simulink model "gimbal_model_dynamics_kinematics_test_250120"  (R2018b)
settings: Solver=VariableStepAuto  StartTime=0.0  StopTime=10.0  RelTol=1e-3
values from neighbouring files (symbols this model uses):
  DIM = data{4}    [gimbal_dynamics.m]
  DIS = data{5}    [gimbal_dynamics.m]
  I1 = data{1}    [gimbal_dynamics.m]    (also in macierze_inercji.m = sym('I1', [4 4]))
  I2 = data{2}    [gimbal_dynamics.m]    (also in macierze_inercji.m = sym('I2', [4 4]))
  I3 = data{3}    [gimbal_dynamics.m]    (also in macierze_inercji.m = sym('I3', [4 4]))
  M = [ud_ucz(3:p-1) ud_ucz(3:p-1).^2 ud_ucz(3:p-1).^3 ud_ucz(2:p-2) ud_ucz(2:p-2).^2 ud_ucz(2:p-2).^3 ud_ucz(1:p-3) ud_ucz(1:p-3).^2 ud_ucz(1:p-3).^3 yd_ucz(3:p-1) yd_ucz(3:p-1).^2 yd_ucz(3:p-1).^3 yd_ucz(2:p-2) yd_ucz(2:p-2).^2 yd_ucz(2:p-2).^3 yd_ucz(1:p-3) yd_ucz(1:p-3).^2 yd_ucz(1:p-3).^3]    [Identification_20191023.m]    (also in MI_beta.m = fillmissing(M,'spline'); gimbal_dynamics.m = data{6}; macierze_inercji.m = sym('M', [1 3]))
libraries: robotcorelib x5
settings Model: Creator=Paweł Tymiński  LastModifiedBy=Paweł Tymiński

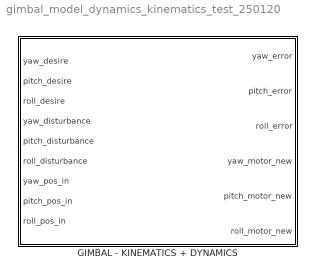
== system gimbal_model_dynamics_kinematics_test_250120 ==
  GIMBAL - KINEMATICS + DYNAMICS : Subsystem

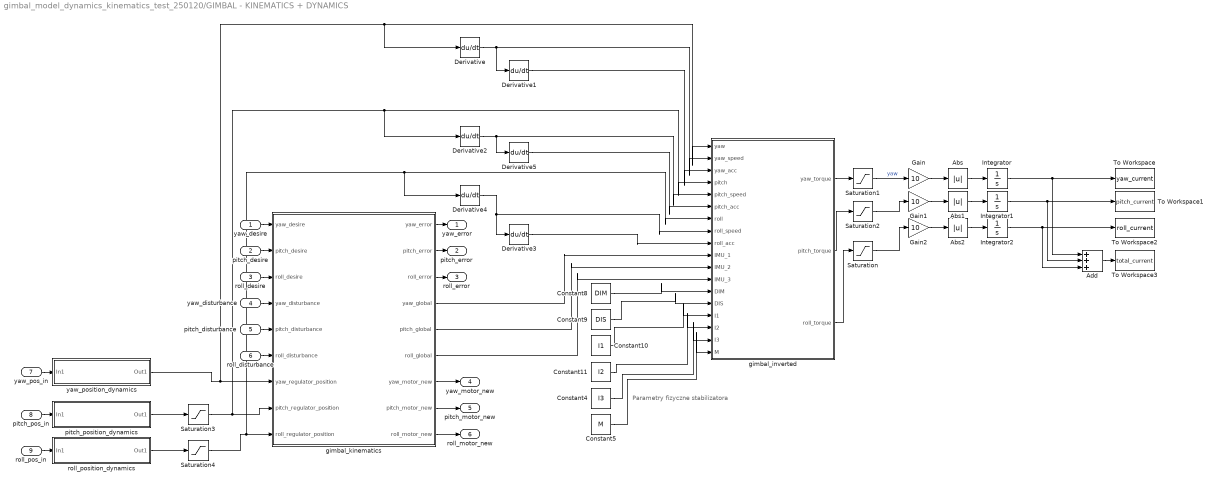
== system gimbal_model_dynamics_kinematics_test_250120/GIMBAL - KINEMATICS + DYNAMICS ==
  note: Parametry fizyczne stabilizatora
  yaw_desire : Inport
  pitch_desire : Inport  Port=2
  roll_desire : Inport  Port=3
  yaw_disturbance : Inport  Port=4
  pitch_disturbance : Inport  Port=5
  roll_disturbance : Inport  Port=6
  yaw_pos_in : Inport  Port=7
  pitch_pos_in : Inport  Port=8
  roll_pos_in : Inport  Port=9
  Abs : Abs
  Abs1 : Abs
  Abs2 : Abs
  Add : Sum  Inputs=+++
  Constant10 : Constant  Value=I1
  Constant11 : Constant  Value=I2
  Constant4 : Constant  Value=I3
  Constant5 : Constant  Value=M
  Constant8 : Constant  Value=DIM
  Constant9 : Constant  Value=DIS
  Derivative{,1..5} (6 alike) : Derivative
  Gain : Gain  Gain=10
  Gain1 : Gain  Gain=10
  Gain2 : Gain  Gain=10
  Integrator : Integrator
  Integrator1 : Integrator
  Integrator2 : Integrator
  Saturation : Saturate  UpperLimit=0.34  LowerLimit=-0.34
  Saturation1 : Saturate  UpperLimit=0.34  LowerLimit=-.34
  Saturation2 : Saturate  UpperLimit=0.34  LowerLimit=-0.34
  Saturation3 : Saturate  UpperLimit=2.35  LowerLimit=-2.35
  Saturation4 : Saturate  UpperLimit=3.84  LowerLimit=-3.84
  To Workspace : ToWorkspace  VariableName=yaw_current  SaveFormat=Timeseries  SampleTime=-1
  To Workspace1 : ToWorkspace  VariableName=pitch_current  SaveFormat=Timeseries  SampleTime=-1
  To Workspace2 : ToWorkspace  VariableName=roll_current  SaveFormat=Timeseries  SampleTime=-1
  To Workspace3 : ToWorkspace  VariableName=total_current  SaveFormat=Timeseries  SampleTime=-1
  gimbal_inverted : MATLAB Function  TreatAsAtomicUnit=on
  gimbal_kinematics : Subsystem
  pitch_position_dynamics : Subsystem
  roll_position_dynamics : Subsystem
  yaw_position_dynamics : Subsystem
  yaw_error : Outport
  pitch_error : Outport  Port=2
  roll_error : Outport  Port=3
  yaw_motor_new : Outport  Port=4
  pitch_motor_new : Outport  Port=5
  roll_motor_new : Outport  Port=6
  wires:
  Constant9/1 -> gimbal_inverted/14(DIS)
  Abs/1 -> Integrator/1
  Derivative5/1 -> gimbal_inverted/6(pitch_acc)
  gimbal_kinematics/3(roll_error) -> roll_error/1
  Gain/1 -> Abs/1
  Abs2/1 -> Integrator2/1
  pitch_desire/1 -> gimbal_kinematics/2(pitch_desire)
  yaw_position_dynamics/1(Out1) -> Derivative/1, gimbal_inverted/1(yaw), gimbal_kinematics/7(yaw_regulator_position)
  gimbal_kinematics/9(roll_motor_new) -> roll_motor_new/1
  Saturation4/1 -> Derivative4/1, gimbal_inverted/7(roll), gimbal_kinematics/9(roll_regulator_position)
  Abs1/1 -> Integrator1/1
  Integrator/1 -> Add/1, To Workspace/1
  roll_pos_in/1 -> roll_position_dynamics/1(In1)
  Saturation1/1 -> Gain/1  "yaw"
  Integrator1/1 -> Add/2, To Workspace1/1
  Gain2/1 -> Abs2/1
  Constant10/1 -> gimbal_inverted/15(I1)
  Derivative2/1 -> gimbal_inverted/5(pitch_speed), Derivative5/1
  Gain1/1 -> Abs1/1
  gimbal_inverted/2(pitch_torque) -> Saturation2/1
  Derivative1/1 -> gimbal_inverted/3(yaw_acc)
  Integrator2/1 -> Add/3, To Workspace2/1
  Constant11/1 -> gimbal_inverted/16(I2)
  Saturation/1 -> Gain2/1
  roll_desire/1 -> gimbal_kinematics/3(roll_desire)
  yaw_disturbance/1 -> gimbal_kinematics/4(yaw_disturbance)
  Derivative/1 -> Derivative1/1, gimbal_inverted/2(yaw_speed)
  Saturation2/1 -> Gain1/1
  roll_position_dynamics/1(Out1) -> Saturation4/1
  Constant5/1 -> gimbal_inverted/18(M)
  gimbal_inverted/1(yaw_torque) -> Saturation1/1
  gimbal_kinematics/6(roll_global) -> gimbal_inverted/12(IMU_3)
  Derivative4/1 -> Derivative3/1, gimbal_inverted/8(roll_speed)
  roll_disturbance/1 -> gimbal_kinematics/6(roll_disturbance)
  gimbal_inverted/3(roll_torque) -> Saturation/1
  gimbal_kinematics/7(yaw_motor_new) -> yaw_motor_new/1
  yaw_pos_in/1 -> yaw_position_dynamics/1(In1)
  Constant4/1 -> gimbal_inverted/17(I3)
  Constant8/1 -> gimbal_inverted/13(DIM)
  Saturation3/1 -> Derivative2/1, gimbal_inverted/4(pitch), gimbal_kinematics/8(pitch_regulator_position)
  Derivative3/1 -> gimbal_inverted/9(roll_acc)
  pitch_position_dynamics/1(Out1) -> Saturation3/1
  gimbal_kinematics/5(pitch_global) -> gimbal_inverted/11(IMU_2)
  gimbal_kinematics/4(yaw_global) -> gimbal_inverted/10(IMU_1)
  gimbal_kinematics/1(yaw_error) -> yaw_error/1
  Add/1 -> To Workspace3/1
  pitch_disturbance/1 -> gimbal_kinematics/5(pitch_disturbance)
  gimbal_kinematics/2(pitch_error) -> pitch_error/1
  gimbal_kinematics/8(pitch_motor_new) -> pitch_motor_new/1
  pitch_pos_in/1 -> pitch_position_dynamics/1(In1)
  yaw_desire/1 -> gimbal_kinematics/1(yaw_desire)

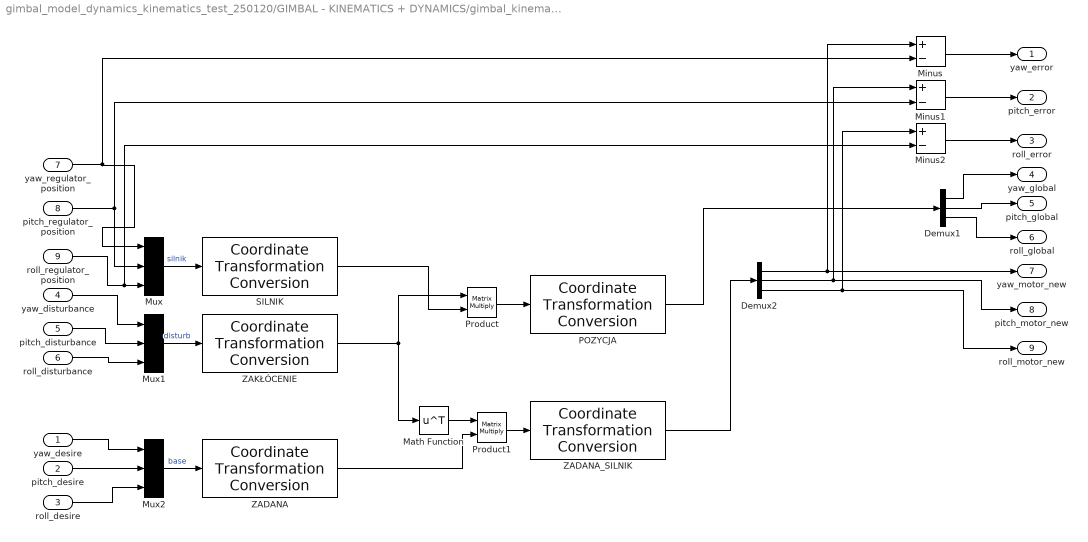
== system gimbal_model_dynamics_kinematics_test_250120/GIMBAL - KINEMATICS + DYNAMICS/gimbal_kinematics ==
  yaw_desire : Inport
  pitch_desire : Inport  Port=2
  roll_desire : Inport  Port=3
  yaw_disturbance : Inport  Port=4
  pitch_disturbance : Inport  Port=5
  roll_disturbance : Inport  Port=6
  yaw_regulator_position : Inport  Port=7
  pitch_regulator_position : Inport  Port=8
  roll_regulator_position : Inport  Port=9
  Demux1 : Demux  Outputs=3
  Demux2 : Demux  Outputs=3
  Math Function : Math  Operator=transpose  SaturateOnIntegerOverflow=on
  Minus : Sum  Inputs=+-
  Minus1 : Sum  Inputs=+-
  Minus2 : Sum  Inputs=+-
  Mux : Mux  Inputs=3
  Mux1 : Mux  Inputs=3
  Mux2 : Mux  Inputs=3
  POZYCJA : robotcorelib/Coordinate Transformation Conversion  InputRepresentation=Rotation Matrix  InputEulerSequence=ZYX  ShowTrVecInputPort=on  OutputRepresentation=Euler Angles  OutputEulerSequence=ZYX  ShowTrVecOutputPort=on  SimulateUsing=Interpreted execution
      settings: SourceProductBaseCode=RO
  Product : Product  Multiplication=Matrix(*)
  Product1 : Product  Multiplication=Matrix(*)
  SILNIK : robotcorelib/Coordinate Transformation Conversion  InputRepresentation=Euler Angles  InputEulerSequence=ZYX  ShowTrVecInputPort=on  OutputRepresentation=Rotation Matrix  OutputEulerSequence=ZYX  ShowTrVecOutputPort=on  SimulateUsing=Interpreted execution
      settings: SourceProductBaseCode=RO
  ZADANA : robotcorelib/Coordinate Transformation Conversion  InputRepresentation=Euler Angles  InputEulerSequence=ZYX  ShowTrVecInputPort=on  OutputRepresentation=Rotation Matrix  OutputEulerSequence=ZYX  ShowTrVecOutputPort=on  SimulateUsing=Interpreted execution
      settings: SourceProductBaseCode=RO
  ZADANA_SILNIK : robotcorelib/Coordinate Transformation Conversion  InputRepresentation=Rotation Matrix  InputEulerSequence=ZYX  ShowTrVecInputPort=on  OutputRepresentation=Euler Angles  OutputEulerSequence=ZYX  ShowTrVecOutputPort=on  SimulateUsing=Interpreted execution
      settings: SourceProductBaseCode=RO
  ZAKŁÓCENIE : robotcorelib/Coordinate Transformation Conversion  InputRepresentation=Euler Angles  InputEulerSequence=ZYX  ShowTrVecInputPort=on  OutputRepresentation=Rotation Matrix  OutputEulerSequence=ZYX  ShowTrVecOutputPort=on  SimulateUsing=Interpreted execution
      settings: SourceProductBaseCode=RO
  yaw_error : Outport
  pitch_error : Outport  Port=2
  roll_error : Outport  Port=3
  yaw_global : Outport  Port=4
  pitch_global : Outport  Port=5
  roll_global : Outport  Port=6
  yaw_motor_new : Outport  Port=7
  pitch_motor_new : Outport  Port=8
  roll_motor_new : Outport  Port=9
  wires:
  ZADANA_SILNIK/1 -> Demux2/1
  ZADANA/1 -> Product1/2
  Product/1 -> POZYCJA/1
  Mux1/1 -> ZAKŁÓCENIE/1  "disturb"
  SILNIK/1 -> Product/2
  Math Function/1 -> Product1/1
  Product1/1 -> ZADANA_SILNIK/1
  Mux/1 -> SILNIK/1  "silnik"
  Mux2/1 -> ZADANA/1  "base"
  ZAKŁÓCENIE/1 -> Math Function/1, Product/1
  pitch_desire/1 -> Mux2/2
  yaw_desire/1 -> Mux2/1
  roll_desire/1 -> Mux2/3
  yaw_disturbance/1 -> Mux1/1
  pitch_disturbance/1 -> Mux1/2
  roll_disturbance/1 -> Mux1/3
  roll_regulator_position/1 -> Mux/3, Minus2/2
  pitch_regulator_position/1 -> Mux/2, Minus1/2
  yaw_regulator_position/1 -> Mux/1, Minus/2
  Demux1/2 -> pitch_global/1
  Demux1/1 -> yaw_global/1
  Demux1/3 -> roll_global/1
  Demux2/1 -> Minus/1, yaw_motor_new/1
  Demux2/2 -> Minus1/1, pitch_motor_new/1
  Demux2/3 -> Minus2/1, roll_motor_new/1
  Minus/1 -> yaw_error/1
  POZYCJA/1 -> Demux1/1
  Minus1/1 -> pitch_error/1
  Minus2/1 -> roll_error/1

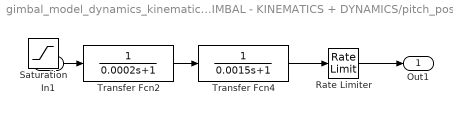
== system gimbal_model_dynamics_kinematics_test_250120/GIMBAL - KINEMATICS + DYNAMICS/pitch_position_dynamics ==
  In1 : Inport
  Rate Limiter : RateLimiter  RisingSlewLimit=18.5  FallingSlewLimit=-18.5  SampleTimeMode=inherited
  Saturation : Saturate  UpperLimit=58.5  LowerLimit=-58.5
  Transfer Fcn2 : TransferFcn  Denominator=[0.0002 1]
  Transfer Fcn4 : TransferFcn  Denominator=[0.0015 1]
  Out1 : Outport
  wires:
  Transfer Fcn2/1 -> Transfer Fcn4/1
  In1/1 -> Transfer Fcn2/1
  Transfer Fcn4/1 -> Rate Limiter/1
  Rate Limiter/1 -> Out1/1

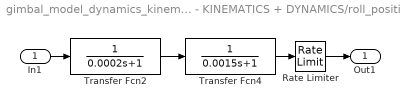
== system gimbal_model_dynamics_kinematics_test_250120/GIMBAL - KINEMATICS + DYNAMICS/roll_position_dynamics ==
  In1 : Inport
  Rate Limiter : RateLimiter  RisingSlewLimit=18.5  FallingSlewLimit=-18.5  SampleTimeMode=inherited
  Transfer Fcn2 : TransferFcn  Denominator=[0.0002 1]
  Transfer Fcn4 : TransferFcn  Denominator=[0.0015 1]
  Out1 : Outport
  wires:
  Transfer Fcn2/1 -> Transfer Fcn4/1
  In1/1 -> Transfer Fcn2/1
  Transfer Fcn4/1 -> Rate Limiter/1
  Rate Limiter/1 -> Out1/1

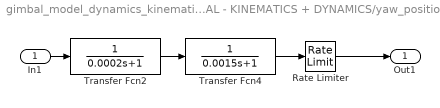
== system gimbal_model_dynamics_kinematics_test_250120/GIMBAL - KINEMATICS + DYNAMICS/yaw_position_dynamics ==
  In1 : Inport
  Rate Limiter : RateLimiter  RisingSlewLimit=18.5  FallingSlewLimit=-18.5  SampleTimeMode=inherited
  Transfer Fcn2 : TransferFcn  Denominator=[0.0002 1]
  Transfer Fcn4 : TransferFcn  Denominator=[0.0015 1]
  Out1 : Outport
  wires:
  Transfer Fcn2/1 -> Transfer Fcn4/1
  In1/1 -> Transfer Fcn2/1
  Transfer Fcn4/1 -> Rate Limiter/1
  Rate Limiter/1 -> Out1/1

== matlab function gimbal_model_dynamics_kinematics_test_250120/GIMBAL - KINEMATICS + DYNAMICS/gimbal_inverted ==
  data: yaw input; yaw_speed input; yaw_acc input; pitch input; pitch_speed input; pitch_acc input; roll input; yaw_torque output; roll_speed input; roll_acc input; IMU_1 input; IMU_2 input; IMU_3 input; DIM input; DIS input; I1 input; I2 input; I3 input; M input; pitch_torque output; roll_torque output
function [yaw_torque, pitch_torque, roll_torque]  = gimbal_dynamics(yaw,yaw_speed,yaw_acc,pitch,pitch_speed,pitch_acc,roll,roll_speed, roll_acc,IMU_1,IMU_2,IMU_3,DIM,DIS,I1,I2,I3,M)

%stała grawitacji
g = 9.81;


%-------------ZMIENNE--------------
% odczyty z IMU
alpha_1 = IMU_1;
alpha_2 = IMU_2;
alpha_3 = IMU_3;
IMU = [alpha_1; alpha_2; alpha_3];
%predkosci katowe osiagane przez gimbal
 om_1 = yaw_speed ;
 om_2 = pitch_speed ;
 om_3 = roll_speed ;
Omega = [om_1; om_2; om_3];
%kąty osiagane aktualnie przez gimbal
 theta_1 = yaw ;
 theta_2 = pitch ;
 theta_3 = roll ;
 THETA = [theta_1; theta_2; theta_3];
% przyśpieszenia kątowe w osiach gimbala
 ACC = [yaw_acc;pitch_acc;roll_acc];

%---------------FUNKCJE---------------------

H = calculate_H_matrix(THETA,Omega,I1,I2,I3,DIM);
D = calculate_D_matrix(THETA,I1,I2,I3,DIM);
G = calculate_G_matrix(IMU,THETA,DIM,g,M,DIS);
Q = D*ACC+H+G;
yaw_torque = Q(1);
pitch_torque = Q(2);
roll_torque = Q(3);

end
